simulink model "luenberger"  (R2019b)
settings: Solver=VariableStepAuto  StartTime=0.0  StopTime=20.0  RelTol=1e-3
libraries: cstblocks x1
settings Model: Creator=jgakl

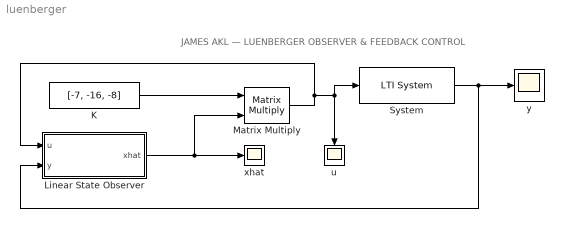
== system luenberger ==
  note: JAMES AKL — LUENBERGER OBSERVER & FEEDBACK CONTROL
  K : Constant  Value=[-7, -16, -8]  VectorParams1D=off
  Linear State Observer : Subsystem
  Matrix Multiply : Product  Multiplication=Matrix(*)
  System : cstblocks/LTI System  sys=ss([0 1 0; 0 1 1; 1 -2 1],[0;0;1],[0 0 1],0)  IC=[0;0;0]
  u : Scope
  xhat : Scope
  y : Scope
  wires:
  System/1 -> Linear State Observer/2(y), y/1
  K/1 -> Matrix Multiply/1
  Matrix Multiply/1 -> u/1, System/1, Linear State Observer/1(u)
  Linear State Observer/1(xhat) -> Matrix Multiply/2, xhat/1

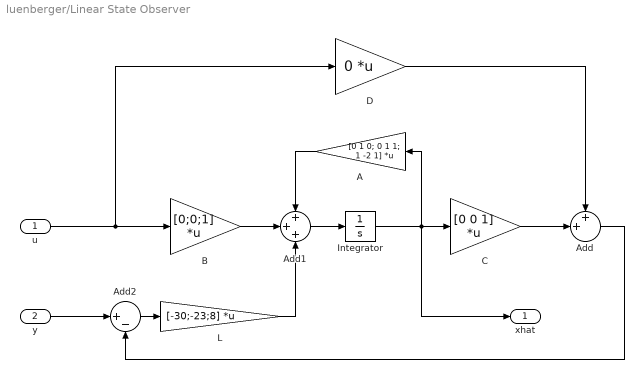
== system luenberger/Linear State Observer ==
  u : Inport
  y : Inport  Port=2
  A : Gain  Gain=[0 1 0; 0 1 1; 1 -2 1]  Multiplication=Matrix(K*u) (u vector)
  Add : Sum  Inputs=++|
  Add1 : Sum  Inputs=+++
  Add2 : Sum  Inputs=|+-
  B : Gain  Gain=[0;0;1]  Multiplication=Matrix(K*u) (u vector)
  C : Gain  Gain=[0 0 1]  Multiplication=Matrix(K*u) (u vector)
  D : Gain  Gain=0  Multiplication=Matrix(K*u) (u vector)
  Integrator : Integrator  InitialCondition=[1 2 3]
  L : Gain  Gain=[-30;-23;8]  Multiplication=Matrix(K*u) (u vector)
  xhat : Outport
  wires:
  u/1 -> D/1, B/1
  D/1 -> Add/1
  B/1 -> Add1/2
  Add1/1 -> Integrator/1
  C/1 -> Add/2
  Add/1 -> Add2/2
  A/1 -> Add1/1
  y/1 -> Add2/1
  Add2/1 -> L/1
  L/1 -> Add1/3
  Integrator/1 -> xhat/1, A/1, C/1
